simulink model "SignalGenerator"  (R2026a)
settings: Solver=VariableStepAuto  StartTime=0  StopTime=5e-5  MaxStep=5e-12  RelTol=1e-8
values from neighbouring files (symbols this model uses):
  ImTable = zeros(N,1)    [suggestion.m]
  RealTable = zeros(N,1)    [suggestion.m]
libraries: hdlsllib x1, dsphdlxfrm2 x1
settings Model: Creator=adams  LastModifiedBy=adams
settings OptimizationCC: ConditionallyExecuteInputs=off
settings SimscapeCC: SimscapeNominalValues="[{\"value\":\"1\",\"unit\":\"A\"},{\"value\":\"1\",\"unit\":\"bar\"},{\"value\":\"1\",\"unit\":\"cm^2\"},{\"value\":\"1\",\"unit\":\"cm^3/s\"},{\"value\":\"1\",\"unit\":\"kJ/kg\"},{\"value\":\"1\",\"unit\":\"kW\"},{\"value\":\"1\",\"unit\":\"l\"},{\"value\":\"1\",\"unit\":\"N\"},{\"value\":\"1\",\"unit\":\"N*m\"},{\"value\":\"1\",\"unit\":\"V\"}]"  SimscapeLogType=none  SimscapeLogDataHistory=5000.0

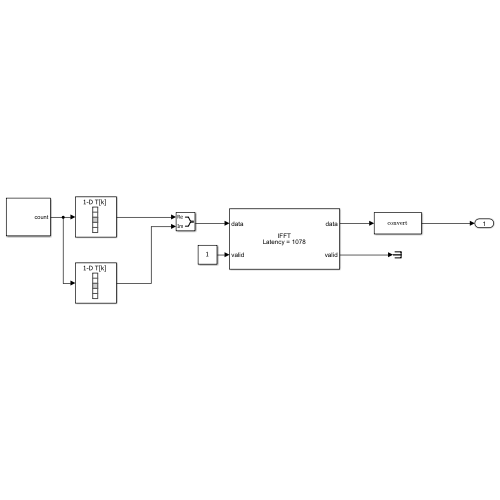
[thumbnail: Simulink's stored preview of the top-level diagram]
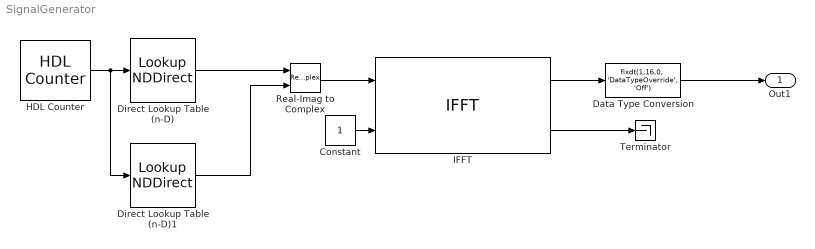
== system SignalGenerator ==
  Constant : Constant  OutDataTypeStr=boolean
  Data Type Conversion : DataTypeConversion  OutDataTypeStr=fixdt(1,16,0, 'DataTypeOverride', 'Off')  RndMeth=Nearest  SaturateOnIntegerOverflow=off
  Direct Lookup Table (n-D) : LookupNDDirect  NumberOfTableDimensions=1  Table=RealTable  TableDataTypeStr=fixdt(1,32,17)
  Direct Lookup Table (n-D)1 : LookupNDDirect  NumberOfTableDimensions=1  Table=ImTable  TableDataTypeStr=fixdt(1,32,17)
  HDL Counter : hdlsllib/Sources/HDL Counter  CountType=Count limited  CountInit=0  CountStep=1  CountMax=511  CountFromType=Initial value  CountFrom=0  CountResetPort=off  CountLoadPort=off  CountEnbPort=off  CountDirPort=off  CountHitOutputPort=off  CountDataType=Unsigned  CountWordLen=9  CountFracLen=0  CountSampTime=1/307200000
  IFFT : dsphdlxfrm2/IFFT  Architecture=Streaming Radix 2^2  FFTLengthSource=Property  FFTLength=512  FFTLengthMax=1024  ComplexMultiplication=Use 3 multipliers and 5 adders  BitReversedOutput=off  BitReversedInput=off  Normalize=off  SimulateUsing=Code generation  RoundingMethod=Nearest  ResetInputPort=off  StartOutputPort=off  EndOutputPort=off
  Real-Imag to Complex : RealImagToComplex
  Terminator : Terminator
  Out1 : Outport
  wires:
  IFFT/2 -> Terminator/1
  HDL Counter/1 -> Direct Lookup Table (n-D)1/1, Direct Lookup Table (n-D)/1
  Constant/1 -> IFFT/2
  Real-Imag to Complex/1 -> IFFT/1
  Direct Lookup Table (n-D)/1 -> Real-Imag to Complex/1
  Direct Lookup Table (n-D)1/1 -> Real-Imag to Complex/2
  IFFT/1 -> Data Type Conversion/1
  Data Type Conversion/1 -> Out1/1
